simulink model "gm_sampleModel1988_sub"  (R2023a)
settings: Solver=VariableStepAuto  StartTime=0.0  StopTime=10.0  RelTol=1e-3
libraries: simulink x4, hdlsllib x2
settings Model: Creator=user1  LastModifiedBy=user1
settings OptimizationCC: BlockReduction=off  ConditionallyExecuteInputs=off
settings DebuggingCC: InheritedTsInSrcMsg=none

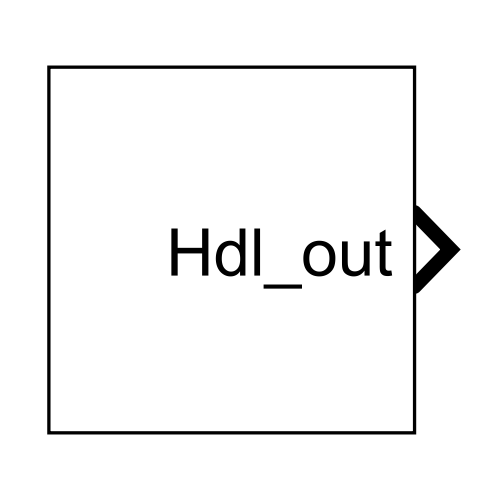
[thumbnail: Simulink's stored preview of the top-level diagram]
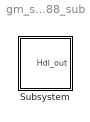
== system gm_sampleModel1988_sub ==
  Subsystem : Subsystem

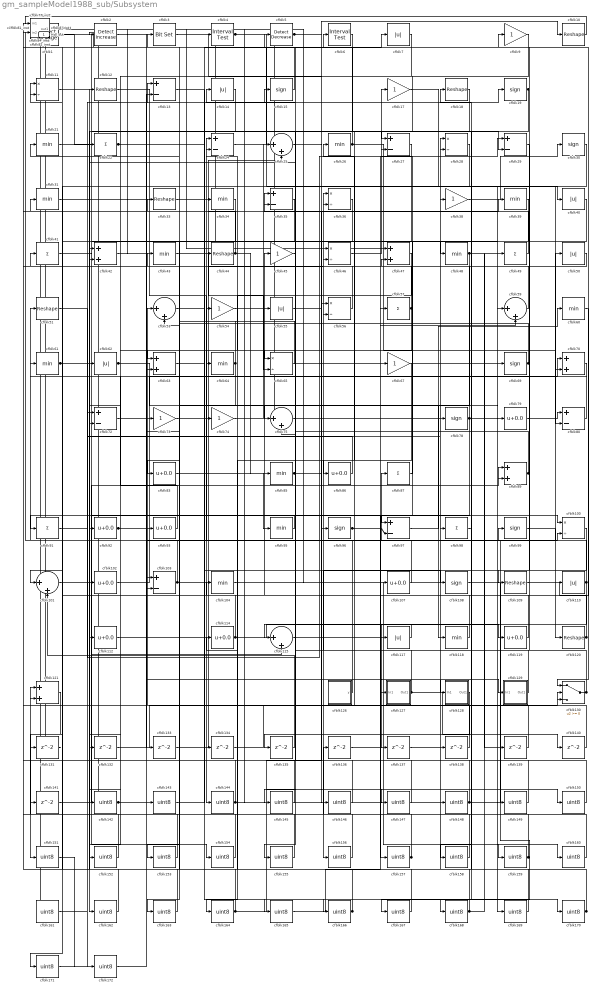
== system gm_sampleModel1988_sub/Subsystem ==
  cfblk1 : simulink/Logic and Bit Operations/Detect Change  vinit=0  OutDataTypeStr=uint8
      settings: LibrarySourceBlock=|
      | hdlsllib/Logic and Bit
      | Operations/Detect
      | Change
  cfblk{10,12,18,33,44,51,109,120} (8 alike) : Reshape
  cfblk{11,28,36,46,56,65,100} (7 alike) : Product  Inputs=*/  OutDataTypeStr=uint8  RndMeth=Zero  SaturateOnIntegerOverflow=on
  cfblk{25,53,59,75,101,115} (6 alike) : Sum  Inputs=|++  OutDataTypeStr=uint8
  cfblk{79,83,86,92..93,102,107,112,114,119} (10 alike) : Bias  Bias=0.0  SaturateOnIntegerOverflow=off
  cfblk{13,24,27,29,35,72,80,97,103} (9 alike) : Sum  Inputs=+-  OutDataTypeStr=uint8
  cfblk{21,26,31,34,39,43,48,60..61,64,85,95,104,118} (14 alike) : MinMax  OutDataTypeStr=uint8
  cfblk{15,19,30,69,78,96,99,108} (8 alike) : Signum
  cfblk{7,14,40,50,55,62,110,117} (8 alike) : Abs  OutDataTypeStr=uint8  SaturateOnIntegerOverflow=off
  cfblk113_inst : Subsystem
  cfblk{42,47,63,70,89,121} (6 alike) : Sum  OutDataTypeStr=uint8
  cfblk123_inst : Subsystem
  cfblk126 : Subsystem  mask(Counter Free-Running){NumBits=double(16), tsamp=double(-1)}
      mask prompts: NumBits "Simulink:masks:NumberOfBits_MP"; tsamp "Simulink:masks:SampleTime_MP"
      mask help: Simulink:masks:CounterFreeRunning_MD
  cfblk127 : Subsystem
  cfblk128 : Subsystem
  cfblk129 : Subsystem
  cfblk130 : Switch  OutDataTypeStr=uint8  SaturateOnIntegerOverflow=off  InputSameDT=off
  cfblk{131..141} (11 alike) : Delay  SampleTime=1
  cfblk{142..172} (31 alike) : DataTypeConversion  OutDataTypeStr=uint8  SaturateOnIntegerOverflow=off  RndMeth=Floor
  cfblk{9,17,38,45,54,67,73..74} (8 alike) : Gain  OutDataTypeStr=uint8
  cfblk2 : simulink/Logic and Bit Operations/Detect Increase  vinit=0.0  OutDataTypeStr=uint8
      settings: LibrarySourceBlock=|
      | hdlsllib/Logic and Bit
      | Operations/Detect
      | Increase
  cfblk{22,41,49,57,87,91,98} (7 alike) : Sum  Inputs=+  OutDataTypeStr=uint8
  cfblk3 : simulink/Logic and Bit Operations/Bit Set  iBit=0
      settings: LibrarySourceBlock=|
      | hdlsllib/Logic and Bit
      | Operations/Bit Set
  cfblk37_inst : Subsystem
  cfblk4 : hdlsllib/Logic and Bit Operations/Interval Test  IntervalClosedRight=on  uplimit=0.5  IntervalClosedLeft=on  lowlimit=-0.5  OutDataTypeStr=uint8
  cfblk5 : simulink/Logic and Bit Operations/Detect Decrease  vinit=0.0  OutDataTypeStr=uint8
      settings: LibrarySourceBlock=|
      | hdlsllib/Logic and Bit
      | Operations/Detect
      | Decrease
  cfblk52_inst : Subsystem
  cfblk6 : hdlsllib/Logic and Bit Operations/Interval Test  IntervalClosedRight=on  uplimit=0.5  IntervalClosedLeft=on  lowlimit=-0.5  OutDataTypeStr=uint8
  cfblk71_inst : Subsystem
  cfblk77_inst : Subsystem
  cfblk81_inst : Subsystem
  cfblk82_inst : Subsystem
  cfblk84_inst : Subsystem
  cfblk8_inst : Subsystem
  Hdl_out : Outport  OutDataTypeStr=uint8  SampleTime=1
  wires:
  cfblk1/1 -> cfblk29/2, cfblk115/2
  cfblk10/1 -> cfblk77_inst/1(in1)
  cfblk100/1 -> cfblk156/1
  cfblk101/1 -> cfblk28/1
  cfblk102/1 -> cfblk70/1
  cfblk103/1 -> cfblk25/2, cfblk123_inst/2(in2)
  cfblk104/1 -> cfblk159/1
  cfblk107/1 -> cfblk87/1
  cfblk108/1 -> cfblk167/1
  cfblk109/1 -> cfblk2/1
  cfblk11/1 -> cfblk154/1
  cfblk110/1 -> cfblk24/1, cfblk137/1
  cfblk112/1 -> cfblk35/1
  cfblk113_inst/1(out1) -> cfblk79/1
  cfblk114/1 -> cfblk53/1, cfblk117/1
  cfblk115/1 -> cfblk99/1
  cfblk117/1 -> cfblk115/1
  cfblk118/1 -> cfblk45/1
  cfblk119/1 -> cfblk18/1
  cfblk12/1 -> cfblk144/1
  cfblk120/1 -> cfblk84_inst/2(in2), cfblk36/1
  cfblk121/1 -> cfblk151/1
  cfblk123_inst/1(out1) -> cfblk143/1
  cfblk126/1(y) -> cfblk51/1
  cfblk127/1(Out1) -> cfblk56/2, cfblk140/1
  cfblk128/1(Out1) -> cfblk135/1
  cfblk129/1(Out1) -> cfblk14/1
  cfblk13/1 -> cfblk170/1
  cfblk130/1 -> cfblk113_inst/2(in2), cfblk9/1
  cfblk131/1 -> cfblk1/1
  cfblk132/1 -> cfblk130/2
  cfblk133/1 -> cfblk46/2
  cfblk134/1 -> cfblk130/3
  cfblk135/1 -> cfblk101/2
  cfblk136/1 -> cfblk29/1
  cfblk137/1 -> cfblk28/2
  cfblk138/1 -> cfblk123_inst/1(in1)
  cfblk139/1 -> cfblk36/2
  cfblk14/1 -> cfblk162/1
  cfblk140/1 -> cfblk103/2
  cfblk141/1 -> cfblk89/1
  cfblk142/1 -> cfblk93/1, cfblk89/2
  cfblk143/1 -> cfblk6/1
  cfblk144/1 -> cfblk77_inst/2(in2), cfblk150/1
  cfblk145/1 -> cfblk12/1
  cfblk146/1 -> cfblk55/1
  cfblk147/1 -> cfblk3/1
  cfblk148/1 -> cfblk50/1, cfblk42/1
  cfblk149/1 -> cfblk8_inst/1(in1)
  cfblk15/1 -> cfblk52_inst/1(in1)
  cfblk150/1 -> cfblk8_inst/2(in2)
  cfblk151/1 -> cfblk172/1
  cfblk152/1 -> cfblk121/1
  cfblk153/1 -> cfblk121/2
  cfblk154/1 -> cfblk52_inst/2(in2)
  cfblk155/1 -> cfblk11/1
  cfblk156/1 -> cfblk11/2
  cfblk157/1 -> cfblk71_inst/1(in1), cfblk37_inst/2(in2), cfblk136/1
  cfblk158/1 -> cfblk41/1
  cfblk159/1 -> cfblk92/1, cfblk24/2
  cfblk160/1 -> cfblk104/1
  cfblk161/1 -> cfblk19/1
  cfblk162/1 -> cfblk81_inst/1(in1)
  cfblk163/1 -> cfblk81_inst/2(in2)
  cfblk164/1 -> cfblk82_inst/2(in2), cfblk56/1
  cfblk165/1 -> cfblk67/1
  cfblk166/1 -> cfblk53/2, cfblk114/1, cfblk141/1
  cfblk167/1 -> cfblk73/1
  cfblk168/1 -> cfblk138/1, cfblk49/1
  cfblk169/1 -> cfblk98/1
  cfblk17/1 -> cfblk40/1
  cfblk170/1 -> cfblk82_inst/1(in1), cfblk112/1
  cfblk171/1 -> cfblk13/1
  cfblk172/1 -> cfblk13/2
  cfblk18/1 -> cfblk155/1
  cfblk19/1 -> cfblk86/1, cfblk158/1
  cfblk2/1 -> cfblk103/1
  cfblk21/1 -> cfblk169/1
  cfblk22/1 -> cfblk108/1, Hdl_out/1
  cfblk24/1 -> cfblk7/1
  cfblk25/1 -> cfblk96/1
  cfblk26/1 -> cfblk84_inst/1(in1), cfblk70/2
  cfblk27/1 -> cfblk63/1
  cfblk28/1 -> cfblk171/1
  cfblk29/1 -> cfblk109/1
  cfblk3/1 -> cfblk146/1
  cfblk30/1 -> cfblk75/2
  cfblk31/1 -> cfblk54/1
  cfblk33/1 -> cfblk74/1
  cfblk34/1 -> cfblk101/1
  cfblk35/1 -> cfblk131/1
  cfblk36/1 -> cfblk83/1
  cfblk37_inst/1(out1) -> cfblk4/1
  cfblk38/1 -> cfblk30/1
  cfblk39/1 -> cfblk75/1
  cfblk4/1 -> cfblk80/2, cfblk59/1
  cfblk40/1 -> cfblk97/1
  cfblk41/1 -> cfblk157/1
  cfblk42/1 -> cfblk133/1
  cfblk43/1 -> cfblk65/2
  cfblk44/1 -> cfblk71_inst/2(in2), cfblk85/1
  cfblk45/1 -> cfblk65/1
  cfblk46/1 -> cfblk17/1
  cfblk47/1 -> cfblk64/1
  cfblk48/1 -> cfblk153/1, cfblk139/1
  cfblk49/1 -> cfblk15/1
  cfblk5/1 -> cfblk147/1, cfblk10/1, cfblk48/1
  cfblk50/1 -> cfblk47/2
  cfblk51/1 -> cfblk102/1
  cfblk52_inst/1(out1) -> cfblk34/1
  cfblk53/1 -> cfblk165/1
  cfblk54/1 -> cfblk38/1
  cfblk55/1 -> cfblk127/1(In1)
  cfblk56/1 -> cfblk113_inst/1(in1)
  cfblk57/1 -> cfblk42/2, cfblk132/1
  cfblk59/1 -> cfblk35/2
  cfblk6/1 -> cfblk142/1
  cfblk60/1 -> cfblk130/1
  cfblk61/1 -> cfblk134/1, cfblk31/1
  cfblk62/1 -> cfblk149/1, cfblk118/1
  cfblk63/1 -> cfblk129/1(In1)
  cfblk64/1 -> cfblk163/1, cfblk43/1
  cfblk65/1 -> cfblk21/1
  cfblk67/1 -> cfblk164/1
  cfblk69/1 -> cfblk37_inst/1(in1), cfblk33/1
  cfblk7/1 -> cfblk72/2
  cfblk70/1 -> cfblk63/2
  cfblk71_inst/1(out1) -> cfblk110/1
  cfblk72/1 -> cfblk128/1(In1)
  cfblk73/1 -> cfblk166/1
  cfblk74/1 -> cfblk25/1
  cfblk75/1 -> cfblk57/1
  cfblk77_inst/1(out1) -> cfblk69/1
  cfblk78/1 -> cfblk160/1, cfblk152/1, cfblk145/1, cfblk5/1
  cfblk79/1 -> cfblk80/1
  cfblk8_inst/1(out1) -> cfblk148/1
  cfblk80/1 -> cfblk61/1
  cfblk81_inst/1(out1) -> cfblk161/1
  cfblk82_inst/1(out1) -> cfblk44/1, cfblk46/1
  cfblk83/1 -> cfblk95/1
  cfblk84_inst/1(out1) -> cfblk47/1
  cfblk85/1 -> cfblk107/1, cfblk39/1
  cfblk86/1 -> cfblk72/1
  cfblk87/1 -> cfblk27/2
  cfblk89/1 -> cfblk22/1, cfblk26/1
  cfblk9/1 -> cfblk27/1
  cfblk91/1 -> cfblk78/1
  cfblk92/1 -> cfblk100/2, cfblk100/1
  cfblk93/1 -> cfblk62/1
  cfblk95/1 -> cfblk91/1
  cfblk96/1 -> cfblk97/2, cfblk59/2, cfblk119/1
  cfblk97/1 -> cfblk60/1
  cfblk98/1 -> cfblk168/1
  cfblk99/1 -> cfblk120/1

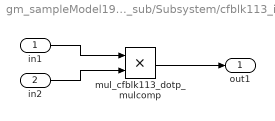
== system gm_sampleModel1988_sub/Subsystem/cfblk113_inst ==
  in1 : Inport  OutDataTypeStr=uint8  SampleTime=1
  in2 : Inport  Port=2  OutDataTypeStr=uint8  SampleTime=1
  mul_cfblk113_dotp_mulcomp : Product  Inputs=**  OutDataTypeStr=uint8  SampleTime=1
  out1 : Outport  OutDataTypeStr=uint8  SampleTime=1
  wires:
  in1/1 -> mul_cfblk113_dotp_mulcomp/1
  in2/1 -> mul_cfblk113_dotp_mulcomp/2
  mul_cfblk113_dotp_mulcomp/1 -> out1/1

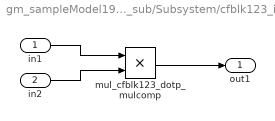
== system gm_sampleModel1988_sub/Subsystem/cfblk123_inst ==
  in1 : Inport  OutDataTypeStr=uint8  SampleTime=1
  in2 : Inport  Port=2  OutDataTypeStr=uint8  SampleTime=1
  mul_cfblk123_dotp_mulcomp : Product  Inputs=**  OutDataTypeStr=uint8  SampleTime=1
  out1 : Outport  OutDataTypeStr=uint8  SampleTime=1
  wires:
  in1/1 -> mul_cfblk123_dotp_mulcomp/1
  in2/1 -> mul_cfblk123_dotp_mulcomp/2
  mul_cfblk123_dotp_mulcomp/1 -> out1/1

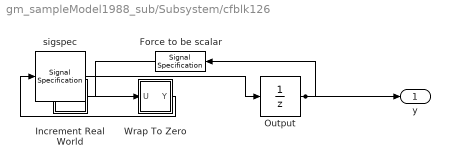
== system gm_sampleModel1988_sub/Subsystem/cfblk126 ==
  Force to be scalar : SignalSpecification  DisableCoverage=on  Dimensions=1
  Increment Real World : Subsystem  mask(Real World Value Increment){}
      mask help: Simulink:masks:RealWorldValueIncrement_MD
      mask Display: disp('V++')
  Output : UnitDelay  InitialCondition=0.0  SampleTime=tsamp  HasFrameUpgradeWarning=on
  Wrap To Zero : Subsystem  mask(Wrap To Zero){Threshold=double(65535)}
      mask prompts: Threshold "Simulink:masks:Threshold_MP"
      mask help: Simulink:masks:WrapToZero_MD
  sigspec : SignalSpecification  OutDataTypeStr=uint16  Dimensions=1
  y : Outport  SampleTime=1
  wires:
  Force to be scalar/1 -> Increment Real World/1(u)
  Increment Real World/1(y) -> Wrap To Zero/1(U)
  Output/1 -> Force to be scalar/1, y/1
  Wrap To Zero/1(Y) -> sigspec/1
  sigspec/1 -> Output/1

== system gm_sampleModel1988_sub/Subsystem/cfblk127 ==
  In1 : Inport  OutDataTypeStr=uint8  PortDimensions=1  SampleTime=1
  Out1 : Outport  SampleTime=1
  wires:
  In1/1 -> Out1/1

== system gm_sampleModel1988_sub/Subsystem/cfblk128 ==
  In1 : Inport  OutDataTypeStr=uint8  PortDimensions=1  SampleTime=1
  Out1 : Outport  SampleTime=1
  wires:
  In1/1 -> Out1/1

== system gm_sampleModel1988_sub/Subsystem/cfblk129 ==
  In1 : Inport  OutDataTypeStr=uint8  PortDimensions=1  SampleTime=1
  Out1 : Outport  SampleTime=1
  wires:
  In1/1 -> Out1/1

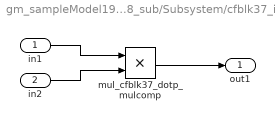
== system gm_sampleModel1988_sub/Subsystem/cfblk37_inst ==
  in1 : Inport  OutDataTypeStr=uint8  SampleTime=1
  in2 : Inport  Port=2  OutDataTypeStr=uint8  SampleTime=1
  mul_cfblk37_dotp_mulcomp : Product  Inputs=**  OutDataTypeStr=uint8  SampleTime=1
  out1 : Outport  OutDataTypeStr=uint8  SampleTime=1
  wires:
  in1/1 -> mul_cfblk37_dotp_mulcomp/1
  in2/1 -> mul_cfblk37_dotp_mulcomp/2
  mul_cfblk37_dotp_mulcomp/1 -> out1/1

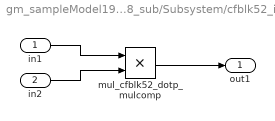
== system gm_sampleModel1988_sub/Subsystem/cfblk52_inst ==
  in1 : Inport  OutDataTypeStr=uint8  SampleTime=1
  in2 : Inport  Port=2  OutDataTypeStr=uint8  SampleTime=1
  mul_cfblk52_dotp_mulcomp : Product  Inputs=**  OutDataTypeStr=uint8  SampleTime=1
  out1 : Outport  OutDataTypeStr=uint8  SampleTime=1
  wires:
  in1/1 -> mul_cfblk52_dotp_mulcomp/1
  in2/1 -> mul_cfblk52_dotp_mulcomp/2
  mul_cfblk52_dotp_mulcomp/1 -> out1/1

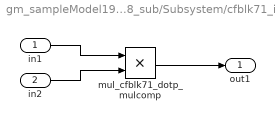
== system gm_sampleModel1988_sub/Subsystem/cfblk71_inst ==
  in1 : Inport  OutDataTypeStr=uint8  SampleTime=1
  in2 : Inport  Port=2  OutDataTypeStr=uint8  SampleTime=1
  mul_cfblk71_dotp_mulcomp : Product  Inputs=**  OutDataTypeStr=uint8  SampleTime=1
  out1 : Outport  OutDataTypeStr=uint8  SampleTime=1
  wires:
  in1/1 -> mul_cfblk71_dotp_mulcomp/1
  in2/1 -> mul_cfblk71_dotp_mulcomp/2
  mul_cfblk71_dotp_mulcomp/1 -> out1/1

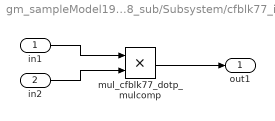
== system gm_sampleModel1988_sub/Subsystem/cfblk77_inst ==
  in1 : Inport  OutDataTypeStr=uint8  SampleTime=1
  in2 : Inport  Port=2  OutDataTypeStr=uint8  SampleTime=1
  mul_cfblk77_dotp_mulcomp : Product  Inputs=**  OutDataTypeStr=uint8  SampleTime=1
  out1 : Outport  OutDataTypeStr=uint8  SampleTime=1
  wires:
  in1/1 -> mul_cfblk77_dotp_mulcomp/1
  in2/1 -> mul_cfblk77_dotp_mulcomp/2
  mul_cfblk77_dotp_mulcomp/1 -> out1/1

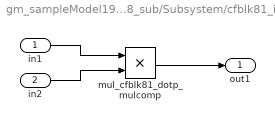
== system gm_sampleModel1988_sub/Subsystem/cfblk81_inst ==
  in1 : Inport  OutDataTypeStr=uint8  SampleTime=1
  in2 : Inport  Port=2  OutDataTypeStr=uint8  SampleTime=1
  mul_cfblk81_dotp_mulcomp : Product  Inputs=**  OutDataTypeStr=uint8  SampleTime=1
  out1 : Outport  OutDataTypeStr=uint8  SampleTime=1
  wires:
  in1/1 -> mul_cfblk81_dotp_mulcomp/1
  in2/1 -> mul_cfblk81_dotp_mulcomp/2
  mul_cfblk81_dotp_mulcomp/1 -> out1/1

== system gm_sampleModel1988_sub/Subsystem/cfblk82_inst ==
  in1 : Inport  OutDataTypeStr=uint8  SampleTime=1
  in2 : Inport  Port=2  OutDataTypeStr=uint8  SampleTime=1
  mul_cfblk82_dotp_mulcomp : Product  Inputs=**  OutDataTypeStr=uint8  SampleTime=1
  out1 : Outport  OutDataTypeStr=uint8  SampleTime=1
  wires:
  in1/1 -> mul_cfblk82_dotp_mulcomp/1
  in2/1 -> mul_cfblk82_dotp_mulcomp/2
  mul_cfblk82_dotp_mulcomp/1 -> out1/1

== system gm_sampleModel1988_sub/Subsystem/cfblk84_inst ==
  in1 : Inport  OutDataTypeStr=uint8  SampleTime=1
  in2 : Inport  Port=2  OutDataTypeStr=uint8  SampleTime=1
  mul_cfblk84_dotp_mulcomp : Product  Inputs=**  OutDataTypeStr=uint8  SampleTime=1
  out1 : Outport  OutDataTypeStr=uint8  SampleTime=1
  wires:
  in1/1 -> mul_cfblk84_dotp_mulcomp/1
  in2/1 -> mul_cfblk84_dotp_mulcomp/2
  mul_cfblk84_dotp_mulcomp/1 -> out1/1

== system gm_sampleModel1988_sub/Subsystem/cfblk8_inst ==
  in1 : Inport  OutDataTypeStr=uint8  SampleTime=1
  in2 : Inport  Port=2  OutDataTypeStr=uint8  SampleTime=1
  mul_cfblk8_dotp_mulcomp : Product  Inputs=**  OutDataTypeStr=uint8  SampleTime=1
  out1 : Outport  OutDataTypeStr=uint8  SampleTime=1
  wires:
  in1/1 -> mul_cfblk8_dotp_mulcomp/1
  in2/1 -> mul_cfblk8_dotp_mulcomp/2
  mul_cfblk8_dotp_mulcomp/1 -> out1/1

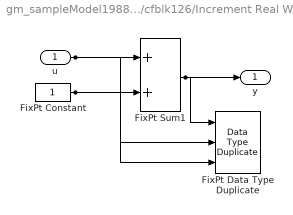
== system gm_sampleModel1988_sub/Subsystem/cfblk126/Increment Real World ==
  u : Inport  OutDataTypeStr=uint16  SampleTime=1
  FixPt Constant : Constant  DisableCoverage=on  OutDataTypeStr=Inherit: Inherit via back propagation  SampleTime=-1
  FixPt Data Type Duplicate : DataTypeDuplicate  DisableCoverage=on  NumInputPorts=3
  FixPt Sum1 : Sum  InputSameDT=on  OutDataTypeStr=Inherit: Inherit via back propagation  LockScale=on
  y : Outport  SampleTime=1
  wires:
  u/1 -> FixPt Sum1/1, FixPt Data Type Duplicate/2
  FixPt Constant/1 -> FixPt Sum1/2, FixPt Data Type Duplicate/3
  FixPt Sum1/1 -> FixPt Data Type Duplicate/1, y/1

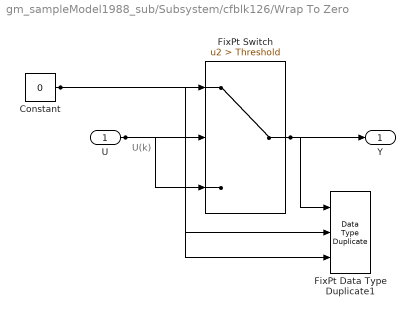
== system gm_sampleModel1988_sub/Subsystem/cfblk126/Wrap To Zero ==
  note: U(k)
  U : Inport  OutDataTypeStr=uint16  SampleTime=1
  Constant : Constant  DisableCoverage=on  Value=0  OutDataTypeStr=Inherit: Inherit via back propagation  SampleTime=-1
  FixPt Data Type Duplicate1 : DataTypeDuplicate  DisableCoverage=on  NumInputPorts=3
  FixPt Switch : Switch  Criteria=u2 > Threshold  Threshold=Threshold  OutDataTypeStr=Inherit: Inherit via back propagation  ZeroCross=off  SaturateOnIntegerOverflow=off  InputSameDT=off
  Y : Outport  SampleTime=1
  wires:
  U/1 -> FixPt Switch/3, FixPt Switch/2, FixPt Data Type Duplicate1/2
  Constant/1 -> FixPt Switch/1, FixPt Data Type Duplicate1/3
  FixPt Switch/1 -> FixPt Data Type Duplicate1/1, Y/1
